simulink model "case33"  (R2014a)
settings: Solver=ode45  StartTime=0.0  StopTime=0.001  RelTol=1e-3
libraries: powerlib x143
(part 1 of 2)
settings Model: Creator=9502085  LastModifiedBy=9502085

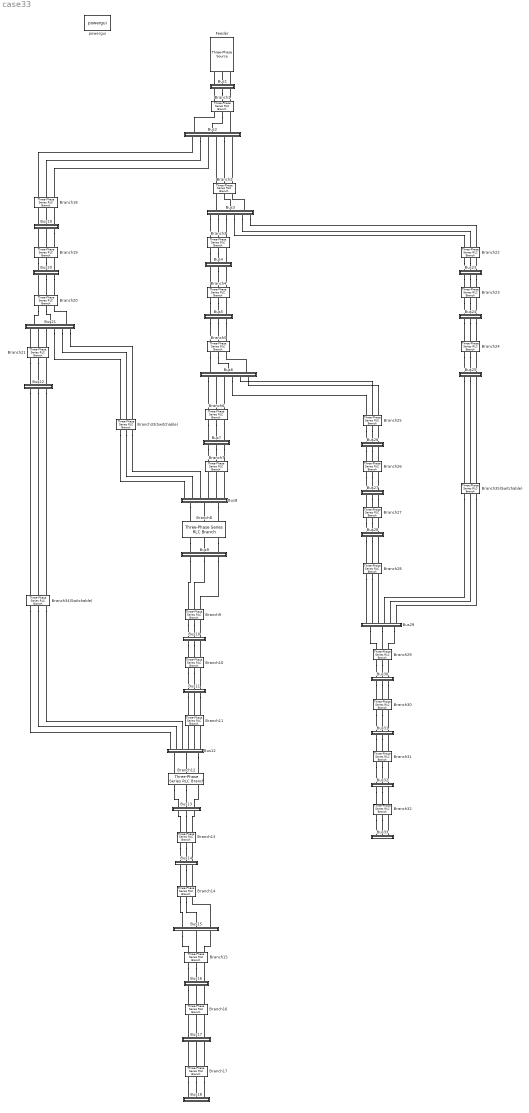
== system case33 ==
  " Branch26" : powerlib/Elements/Three-Phase Series RLC Branch  LConnTagsString=A|B|C  RConnTagsString=A|B|C  BranchType=RLC  Resistance=1  Inductance=1e-3  Capacitance=1e-6  Measurements=None
  Branch{1..25,27..32} (31 alike) : powerlib/Elements/Three-Phase Series RLC Branch  LConnTagsString=A|B|C  RConnTagsString=A|B|C  BranchType=RLC  Resistance=1  Inductance=1e-3  Capacitance=1e-6  Measurements=None
  Branch33(Switchable) : powerlib/Elements/Three-Phase Series RLC Branch  LConnTagsString=A|B|C  RConnTagsString=A|B|C  BranchType=RLC  Resistance=1  Inductance=1e-3  Capacitance=1e-6  Measurements=None
  Branch34(Switchable) : powerlib/Elements/Three-Phase Series RLC Branch  LConnTagsString=A|B|C  RConnTagsString=A|B|C  BranchType=RLC  Resistance=1  Inductance=1e-3  Capacitance=1e-6  Measurements=None
  Branch35(Switchable) : powerlib/Elements/Three-Phase Series RLC Branch  LConnTagsString=A|B|C  RConnTagsString=A|B|C  BranchType=RLC  Resistance=1  Inductance=1e-3  Capacitance=1e-6  Measurements=None
  Bus1 : Subsystem
  Bus10 : Subsystem
  Bus11 : Subsystem
  Bus12 : Subsystem
  Bus13 : Subsystem
  Bus14 : Subsystem
  Bus15 : Subsystem
  Bus16 : Subsystem
  Bus17 : Subsystem
  Bus18 : Subsystem
  Bus19 : Subsystem
  Bus2 : Subsystem
  Bus20 : Subsystem
  Bus21 : Subsystem
  Bus22 : Subsystem
  Bus23 : Subsystem
  Bus24 : Subsystem
  Bus25 : Subsystem
  Bus26 : Subsystem
  Bus27 : Subsystem
  Bus28 : Subsystem
  Bus29 : Subsystem
  Bus3 : Subsystem
  Bus30 : Subsystem
  Bus31 : Subsystem
  Bus32 : Subsystem
  Bus33 : Subsystem
  Bus4 : Subsystem
  Bus5 : Subsystem
  Bus6 : Subsystem
  Bus7 : Subsystem
  Bus8 : Subsystem
  Bus9 : Subsystem
  Feeder : powerlib/Electrical Sources/Three-Phase Source  Voltage=25e3  PhaseAngle=0  Frequency=60  InternalConnection=Yg  SpecifyImpedance=on  Resistance=0.8929  Inductance=16.58e-3  ShortCircuitLevel=100e6  BaseVoltage=25e3  XRratio=7  BusType=swing  Pref=0  Qref=0  Qmin=-inf  Qmax=inf
  powergui : powerlib/powergui  Priority=1  SimulationMode=Continuous  SolverType=Tustin  SampleTime=50e-6  frequency=60  SPID=off  DisableSnubberDevices=off  DisableRonSwitches=off  DisableVfSwitches=off  SwTol=0  Interpol=off  DisplayEquations=off  Ts=0  methode=off  frequencyindice=60  Pbase=100e6  ErrMax=1e-4  Iterations=50  UnitsV=kV  UnitsW=MW  FunctionMessages=off  echomessages=off  HookPort=off  EnableUseOfTLC=off  x0status=blocks  RestoreLinks=warning  ResistiveCurrentMeasurement=off  Frange=[0:2:500]  Ylog=off  Xlog=on  ShowGrid=off  save=off  variable=ZData  structure=0  ZoomFFT=off  StartTime=0.0  cycles=1  DisplayStyle=1  fundamental=60  FreqAxis=off  MaxFrequency=1000  frequencyindicesteady=1  RmsSteady=1  display=off
  connections:
  Bus1/RConn2 -- Branch1/LConn2
  Bus3/RConn2 -- Branch3/LConn2
  Bus3/RConn3 -- Branch3/LConn3
  Bus3/RConn1 -- Branch3/LConn1
  Bus4/RConn2 -- Branch4/LConn2
  Bus5/RConn2 -- Branch5/LConn2
  Bus5/RConn3 -- Branch5/LConn3
  Bus5/RConn1 -- Branch5/LConn1
  Branch6/LConn3 -- Bus6/RConn3
  Bus7/RConn3 -- Branch7/LConn3
  Bus9/RConn1 -- Branch9/LConn1
  Bus19/RConn3 -- Branch19/LConn3
  Bus20/RConn3 -- Branch20/LConn3
  Bus23/RConn3 -- Branch23/LConn3
  Bus27/RConn3 -- Branch27/LConn3
  Bus27/RConn2 -- Branch27/LConn2
  Branch33(Switchable)/RConn1 -- Bus8/LConn1
  Branch33(Switchable)/RConn2 -- Bus8/LConn2
  Branch33(Switchable)/RConn3 -- Bus8/LConn3
  Bus3/LConn1 -- Branch2/RConn1
  Bus3/LConn2 -- Branch2/RConn2
  Bus3/LConn3 -- Branch2/RConn3
  Bus19/LConn3 -- Branch18/RConn3
  Bus19/LConn2 -- Branch18/RConn2
  Bus19/LConn1 -- Branch18/RConn1
  Branch19/LConn1 -- Bus19/RConn1
  Branch19/LConn2 -- Bus19/RConn2
  Bus20/RConn2 -- Branch20/LConn2
  Bus20/LConn3 -- Branch19/RConn3
  Branch19/RConn2 -- Bus20/LConn2
  Branch19/RConn1 -- Bus20/LConn1
  Branch20/LConn1 -- Bus20/RConn1
  Branch20/RConn3 -- Bus21/LConn3
  Branch20/RConn2 -- Bus21/LConn2
  Branch20/RConn1 -- Bus21/LConn1
  Branch21/LConn1 -- Bus21/RConn1
  Branch21/LConn2 -- Bus21/RConn2
  Branch21/LConn3 -- Bus21/RConn3
  Bus22/LConn3 -- Branch21/RConn3
  Branch21/RConn1 -- Bus22/LConn1
  Bus22/RConn1 -- Branch34(Switchable)/LConn1
  Bus22/RConn2 -- Branch34(Switchable)/LConn2
  Bus22/RConn3 -- Branch34(Switchable)/LConn3
  Branch4/LConn3 -- Bus4/RConn3
  Bus4/LConn3 -- Branch3/RConn3
  Branch3/RConn2 -- Bus4/LConn2
  Branch3/RConn1 -- Bus4/LConn1
  Branch4/LConn1 -- Bus4/RConn1
  Bus2/LConn3 -- Branch1/RConn3
  Branch1/RConn2 -- Bus2/LConn2
  Bus2/LConn1 -- Branch1/RConn1
  Bus5/LConn3 -- Branch4/RConn3
  Branch4/RConn2 -- Bus5/LConn2
  Branch4/RConn1 -- Bus5/LConn1
  Bus6/LConn3 -- Branch5/RConn3
  Branch5/RConn2 -- Bus6/LConn2
  Branch5/RConn1 -- Bus6/LConn1
  Bus6/RConn1 -- Branch6/LConn1
  Branch6/LConn2 -- Bus6/RConn2
  Bus7/LConn3 -- Branch6/RConn3
  Branch6/RConn2 -- Bus7/LConn2
  Branch6/RConn1 -- Bus7/LConn1
  Bus7/RConn1 -- Branch7/LConn1
  Bus7/RConn2 -- Branch7/LConn2
  Branch8/RConn3 -- Bus9/LConn3
  Bus9/LConn2 -- Branch8/RConn2
  Branch8/RConn1 -- Bus9/LConn1
  Bus9/RConn2 -- Branch9/LConn2
  Bus9/RConn3 -- Branch9/LConn3
  Bus10/LConn3 -- Branch9/RConn3
  Branch9/RConn2 -- Bus10/LConn2
  Branch9/RConn1 -- Bus10/LConn1
  Bus10/RConn1 -- Branch10/LConn1
  Bus10/RConn2 -- Branch10/LConn2
  Branch10/LConn3 -- Bus10/RConn3
  Bus11/LConn3 -- Branch10/RConn3
  Bus11/RConn3 -- Branch11/LConn3
  Branch11/LConn2 -- Bus11/RConn2
  Bus11/RConn1 -- Branch11/LConn1
  Branch10/RConn1 -- Bus11/LConn1
  Branch10/RConn2 -- Bus11/LConn2
  Bus13/LConn3 -- Branch12/RConn3
  Bus13/RConn3 -- Branch13/LConn3
  Bus13/RConn2 -- Branch13/LConn2
  Branch12/RConn2 -- Bus13/LConn2
  Branch12/RConn1 -- Bus13/LConn1
  Bus13/RConn1 -- Branch13/LConn1
  Bus14/LConn3 -- Branch13/RConn3
  Branch14/LConn3 -- Bus14/RConn3
  Branch13/RConn2 -- Bus14/LConn2
  Branch13/RConn1 -- Bus14/LConn1
  Branch14/LConn1 -- Bus14/RConn1
  Bus14/RConn2 -- Branch14/LConn2
  Bus15/LConn3 -- Branch14/RConn3
  Branch14/RConn2 -- Bus15/LConn2
  Branch14/RConn1 -- Bus15/LConn1
  Bus16/LConn3 -- Branch15/RConn3
  Branch15/RConn2 -- Bus16/LConn2
  Branch15/RConn1 -- Bus16/LConn1
  Bus17/LConn3 -- Branch16/RConn3
  Bus17/LConn2 -- Branch16/RConn2
  Bus17/LConn1 -- Branch16/RConn1
  Branch17/RConn2 -- Bus18/LConn2
  Branch17/RConn1 -- Bus18/LConn1
  Bus23/LConn3 -- Branch22/RConn3
  Branch22/RConn2 -- Bus23/LConn2
  Branch22/RConn1 -- Bus23/LConn1
  Bus23/RConn1 -- Branch23/LConn1
  Bus23/RConn2 -- Branch23/LConn2
  Bus24/LConn3 -- Branch23/RConn3
  Bus24/RConn3 -- Branch24/LConn3
  Branch23/RConn2 -- Bus24/LConn2
  Branch23/RConn1 -- Bus24/LConn1
  Bus24/RConn1 -- Branch24/LConn1
  Bus24/RConn2 -- Branch24/LConn2
  Bus25/LConn3 -- Branch24/RConn3
  Branch35(Switchable)/LConn3 -- Bus25/RConn3
  Bus25/RConn2 -- Branch35(Switchable)/LConn2
  Bus25/RConn1 -- Branch35(Switchable)/LConn1
  Branch24/RConn1 -- Bus25/LConn1
  Branch24/RConn2 -- Bus25/LConn2
  Bus26/LConn3 -- Branch25/RConn3
  " Branch26"/LConn3 -- Bus26/RConn3
  Branch25/RConn2 -- Bus26/LConn2
  Branch25/RConn1 -- Bus26/LConn1
  Bus26/RConn1 -- " Branch26"/LConn1
  Bus26/RConn2 -- " Branch26"/LConn2
  Bus27/LConn3 -- " Branch26"/RConn3
  Branch27/LConn1 -- Bus27/RConn1
  " Branch26"/RConn1 -- Bus27/LConn1
  " Branch26"/RConn2 -- Bus27/LConn2
  Bus28/LConn3 -- Branch27/RConn3
  Branch27/RConn2 -- Bus28/LConn2
  Branch27/RConn1 -- Bus28/LConn1
  Branch28/LConn3 -- Bus28/RConn3
  Bus28/RConn2 -- Branch28/LConn2
  Bus28/RConn1 -- Branch28/LConn1
  Bus29/LConn3 -- Branch28/RConn3
  Branch28/RConn2 -- Bus29/LConn2
  Branch28/RConn1 -- Bus29/LConn1
  Bus29/RConn3 -- Branch29/LConn3
  Bus29/RConn2 -- Branch29/LConn2
  Bus29/RConn1 -- Branch29/LConn1
  Bus30/LConn3 -- Branch29/RConn3
  Branch29/RConn2 -- Bus30/LConn2
  Branch29/RConn1 -- Bus30/LConn1
  Bus30/RConn3 -- Branch30/LConn3
  Bus30/RConn2 -- Branch30/LConn2
  Bus30/RConn1 -- Branch30/LConn1
  Bus31/LConn3 -- Branch30/RConn3
  Branch31/LConn3 -- Bus31/RConn3
  Branch30/RConn2 -- Bus31/LConn2
  Branch30/RConn1 -- Bus31/LConn1
  Bus31/RConn2 -- Branch31/LConn2
  Bus31/RConn1 -- Branch31/LConn1
  Bus32/LConn3 -- Branch31/RConn3
  Branch31/RConn2 -- Bus32/LConn2
  Branch31/RConn1 -- Bus32/LConn1
  Branch32/LConn3 -- Bus32/RConn3
  Bus32/RConn2 -- Branch32/LConn2
  Bus32/RConn1 -- Branch32/LConn1
  Bus33/LConn3 -- Branch32/RConn3
  Branch32/RConn2 -- Bus33/LConn2
  Branch32/RConn1 -- Bus33/LConn1
  Branch17/RConn3 -- Bus18/LConn3
  Bus1/LConn2 -- Feeder/RConn2
  Bus1/LConn1 -- Feeder/RConn1
  Bus1/LConn3 -- Feeder/RConn3
  Branch1/LConn1 -- Bus1/RConn1
  Branch1/LConn3 -- Bus1/RConn3
  Bus6/RConn4 -- Branch25/LConn1
  Bus6/RConn5 -- Branch25/LConn2
  Bus6/RConn6 -- Branch25/LConn3
  Branch2/LConn3 -- Bus2/RConn6
  Bus2/RConn5 -- Branch2/LConn2
  Branch2/LConn1 -- Bus2/RConn4
  Branch18/LConn3 -- Bus2/RConn3
  Bus2/RConn2 -- Branch18/LConn2
  Branch18/LConn1 -- Bus2/RConn1
  Bus3/RConn4 -- Branch22/LConn1
  Bus3/RConn5 -- Branch22/LConn2
  Bus3/RConn6 -- Branch22/LConn3
  Bus8/LConn6 -- Branch7/RConn3
  Bus8/LConn4 -- Branch7/RConn1
  Bus8/LConn5 -- Branch7/RConn2
  Bus8/RConn1 -- Branch8/LConn1
  Branch8/LConn2 -- Bus8/RConn2
  Bus8/RConn3 -- Branch8/LConn3
  Bus21/RConn4 -- Branch33(Switchable)/LConn1
  Bus21/RConn5 -- Branch33(Switchable)/LConn2
  Bus21/RConn6 -- Branch33(Switchable)/LConn3
  Branch21/RConn2 -- Bus22/LConn2
  Bus12/LConn6 -- Branch11/RConn3
  Bus12/LConn5 -- Branch11/RConn2
  Bus12/LConn4 -- Branch11/RConn1
  Branch34(Switchable)/RConn3 -- Bus12/LConn3
  Branch34(Switchable)/RConn2 -- Bus12/LConn2
  Branch34(Switchable)/RConn1 -- Bus12/LConn1
  Branch12/LConn2 -- Bus12/RConn2
  Branch12/LConn1 -- Bus12/RConn1
  Bus12/RConn3 -- Branch12/LConn3
  Branch15/LConn2 -- Bus15/RConn2
  Bus15/RConn1 -- Branch15/LConn1
  Branch15/LConn3 -- Bus15/RConn3
  Branch16/LConn2 -- Bus16/RConn2
  Bus16/RConn1 -- Branch16/LConn1
  Branch16/LConn3 -- Bus16/RConn3
  Branch17/LConn3 -- Bus17/RConn3
  Branch17/LConn2 -- Bus17/RConn2
  Branch17/LConn1 -- Bus17/RConn1
  Branch35(Switchable)/RConn1 -- Bus29/LConn4
  Bus29/LConn5 -- Branch35(Switchable)/RConn2
  Branch35(Switchable)/RConn3 -- Bus29/LConn6

== system case33/Bus1 ==
  Bus1 : powerlib/Measurements/Three-Phase V-I Measurement  VoltageMeasurement=no  SetLabelV=off  LabelV=Vabc  Vpu=off  VpuLL=off  CurrentMeasurement=no  SetLabelI=off  LabelI=Iabc  Ipu=off  Pbase=100e6  Vbase=500e3  OutputType=Complex  PhasorSimulation=off  PSBequivalent=0
  CB1-2 : powerlib/Elements/Three-Phase Breaker  InitialState=open  SwitchA=on  SwitchB=on  SwitchC=on  SwitchTimes="[1/60  5/60]"  External=off  BreakerResistance=0.01  SnubberResistance=1e6  SnubberCapacitance=inf  Measurements=None
  InPhaseA : PMIOPort  Port=1  Side=Left
  InPhaseB : PMIOPort  Port=2  Side=Left
  InPhaseC : PMIOPort  Port=3  Side=Left
  OutPhaseA : PMIOPort  Port=4  Side=Right
  OutPhaseB : PMIOPort  Port=5  Side=Right
  OutPhaseC : PMIOPort  Port=6  Side=Right
  connections:
  CB1-2/LConn1 -- Bus1/RConn1
  CB1-2/RConn3 -- OutPhaseC/RConn1
  CB1-2/LConn2 -- Bus1/RConn2
  CB1-2/LConn3 -- Bus1/RConn3
  CB1-2/RConn1 -- OutPhaseA/RConn1
  CB1-2/RConn2 -- OutPhaseB/RConn1
  InPhaseA/RConn1 -- Bus1/LConn1
  InPhaseB/RConn1 -- Bus1/LConn2
  InPhaseC/RConn1 -- Bus1/LConn3

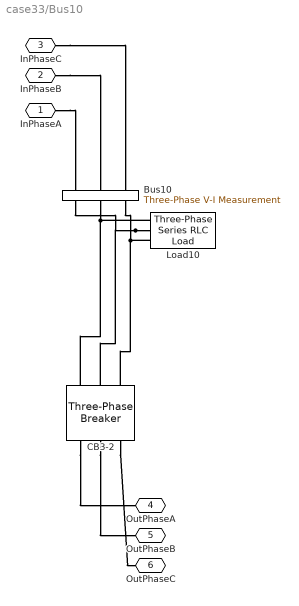
== system case33/Bus10 ==
  Bus10 : powerlib/Measurements/Three-Phase V-I Measurement  VoltageMeasurement=no  SetLabelV=off  LabelV=Vabc  Vpu=off  VpuLL=off  CurrentMeasurement=no  SetLabelI=off  LabelI=Iabc  Ipu=off  Pbase=100e6  Vbase=500e3  OutputType=Complex  PhasorSimulation=off  PSBequivalent=0
  CB3-2 : powerlib/Elements/Three-Phase Breaker  InitialState=open  SwitchA=on  SwitchB=on  SwitchC=on  SwitchTimes="[1/60  5/60]"  External=off  BreakerResistance=0.01  SnubberResistance=1e6  SnubberCapacitance=inf  Measurements=None
  Load10 : powerlib/Elements/Three-Phase Series RLC Load  LConnTagsString=A|B|C  Configuration=Y (grounded)  NominalVoltage=1000  NominalFrequency=60  ActivePower=10e3  InductivePower=100  CapacitivePower=100  Measurements=None  LoadType=constant Z
  InPhaseA : PMIOPort  Port=1  Side=Left
  InPhaseB : PMIOPort  Port=2  Side=Left
  InPhaseC : PMIOPort  Port=3  Side=Left
  OutPhaseA : PMIOPort  Port=4  Side=Right
  OutPhaseB : PMIOPort  Port=5  Side=Right
  OutPhaseC : PMIOPort  Port=6  Side=Right
  connections:
  Bus10/RConn1 -- CB3-2/LConn1 -- Load10/LConn1
  CB3-2/RConn3 -- OutPhaseC/RConn1
  Load10/LConn2 -- CB3-2/LConn2 -- Bus10/RConn2
  Load10/LConn3 -- CB3-2/LConn3 -- Bus10/RConn3
  CB3-2/RConn1 -- OutPhaseA/RConn1
  CB3-2/RConn2 -- OutPhaseB/RConn1
  InPhaseA/RConn1 -- Bus10/LConn1
  InPhaseB/RConn1 -- Bus10/LConn2
  InPhaseC/RConn1 -- Bus10/LConn3

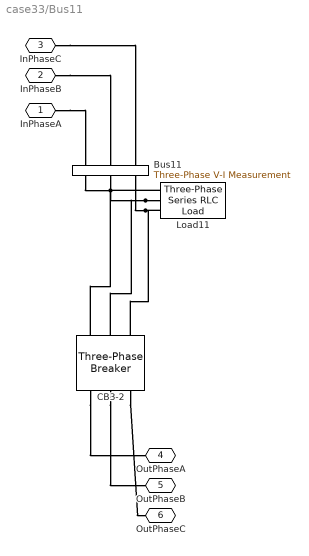
== system case33/Bus11 ==
  Bus11 : powerlib/Measurements/Three-Phase V-I Measurement  VoltageMeasurement=no  SetLabelV=off  LabelV=Vabc  Vpu=off  VpuLL=off  CurrentMeasurement=no  SetLabelI=off  LabelI=Iabc  Ipu=off  Pbase=100e6  Vbase=500e3  OutputType=Complex  PhasorSimulation=off  PSBequivalent=0
  CB3-2 : powerlib/Elements/Three-Phase Breaker  InitialState=open  SwitchA=on  SwitchB=on  SwitchC=on  SwitchTimes="[1/60  5/60]"  External=off  BreakerResistance=0.01  SnubberResistance=1e6  SnubberCapacitance=inf  Measurements=None
  Load11 : powerlib/Elements/Three-Phase Series RLC Load  LConnTagsString=A|B|C  Configuration=Y (grounded)  NominalVoltage=1000  NominalFrequency=60  ActivePower=10e3  InductivePower=100  CapacitivePower=100  Measurements=None  LoadType=constant Z
  InPhaseA : PMIOPort  Port=1  Side=Left
  InPhaseB : PMIOPort  Port=2  Side=Left
  InPhaseC : PMIOPort  Port=3  Side=Left
  OutPhaseA : PMIOPort  Port=4  Side=Right
  OutPhaseB : PMIOPort  Port=5  Side=Right
  OutPhaseC : PMIOPort  Port=6  Side=Right
  connections:
  Bus11/RConn1 -- CB3-2/LConn1 -- Load11/LConn1
  CB3-2/RConn3 -- OutPhaseC/RConn1
  Load11/LConn2 -- CB3-2/LConn2 -- Bus11/RConn2
  Bus11/RConn3 -- CB3-2/LConn3 -- Load11/LConn3
  CB3-2/RConn1 -- OutPhaseA/RConn1
  CB3-2/RConn2 -- OutPhaseB/RConn1
  InPhaseA/RConn1 -- Bus11/LConn1
  InPhaseB/RConn1 -- Bus11/LConn2
  InPhaseC/RConn1 -- Bus11/LConn3

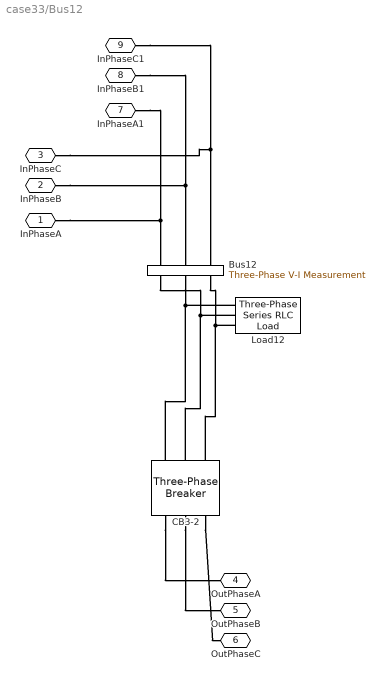
== system case33/Bus12 ==
  Bus12 : powerlib/Measurements/Three-Phase V-I Measurement  VoltageMeasurement=no  SetLabelV=off  LabelV=Vabc  Vpu=off  VpuLL=off  CurrentMeasurement=no  SetLabelI=off  LabelI=Iabc  Ipu=off  Pbase=100e6  Vbase=500e3  OutputType=Complex  PhasorSimulation=off  PSBequivalent=0
  CB3-2 : powerlib/Elements/Three-Phase Breaker  InitialState=open  SwitchA=on  SwitchB=on  SwitchC=on  SwitchTimes="[1/60  5/60]"  External=off  BreakerResistance=0.01  SnubberResistance=1e6  SnubberCapacitance=inf  Measurements=None
  Load12 : powerlib/Elements/Three-Phase Series RLC Load  LConnTagsString=A|B|C  Configuration=Y (grounded)  NominalVoltage=1000  NominalFrequency=60  ActivePower=10e3  InductivePower=100  CapacitivePower=100  Measurements=None  LoadType=constant Z
  InPhaseA : PMIOPort  Port=1  Side=Left
  InPhaseB : PMIOPort  Port=2  Side=Left
  InPhaseC : PMIOPort  Port=3  Side=Left
  OutPhaseA : PMIOPort  Port=4  Side=Right
  OutPhaseB : PMIOPort  Port=5  Side=Right
  OutPhaseC : PMIOPort  Port=6  Side=Right
  InPhaseA1 : PMIOPort  Port=7  Side=Left
  InPhaseB1 : PMIOPort  Port=8  Side=Left
  InPhaseC1 : PMIOPort  Port=9  Side=Left
  connections:
  Load12/LConn1 -- CB3-2/LConn1 -- Bus12/RConn1
  CB3-2/RConn3 -- OutPhaseC/RConn1
  Load12/LConn2 -- CB3-2/LConn2 -- Bus12/RConn2
  Load12/LConn3 -- CB3-2/LConn3 -- Bus12/RConn3
  CB3-2/RConn1 -- OutPhaseA/RConn1
  CB3-2/RConn2 -- OutPhaseB/RConn1
  InPhaseA1/RConn1 -- InPhaseA/RConn1 -- Bus12/LConn1
  InPhaseB1/RConn1 -- InPhaseB/RConn1 -- Bus12/LConn2
  InPhaseC1/RConn1 -- InPhaseC/RConn1 -- Bus12/LConn3

== system case33/Bus13 ==
  Bus13 : powerlib/Measurements/Three-Phase V-I Measurement  VoltageMeasurement=no  SetLabelV=off  LabelV=Vabc  Vpu=off  VpuLL=off  CurrentMeasurement=no  SetLabelI=off  LabelI=Iabc  Ipu=off  Pbase=100e6  Vbase=500e3  OutputType=Complex  PhasorSimulation=off  PSBequivalent=0
  CB3-2 : powerlib/Elements/Three-Phase Breaker  InitialState=open  SwitchA=on  SwitchB=on  SwitchC=on  SwitchTimes="[1/60  5/60]"  External=off  BreakerResistance=0.01  SnubberResistance=1e6  SnubberCapacitance=inf  Measurements=None
  Load13 : powerlib/Elements/Three-Phase Series RLC Load  LConnTagsString=A|B|C  Configuration=Y (grounded)  NominalVoltage=1000  NominalFrequency=60  ActivePower=10e3  InductivePower=100  CapacitivePower=100  Measurements=None  LoadType=constant Z
  InPhaseA : PMIOPort  Port=1  Side=Left
  InPhaseB : PMIOPort  Port=2  Side=Left
  InPhaseC : PMIOPort  Port=3  Side=Left
  OutPhaseA : PMIOPort  Port=4  Side=Right
  OutPhaseB : PMIOPort  Port=5  Side=Right
  OutPhaseC : PMIOPort  Port=6  Side=Right
  connections:
  Load13/LConn1 -- CB3-2/LConn1 -- Bus13/RConn1
  CB3-2/RConn3 -- OutPhaseC/RConn1
  Load13/LConn2 -- CB3-2/LConn2 -- Bus13/RConn2
  Bus13/RConn3 -- CB3-2/LConn3 -- Load13/LConn3
  CB3-2/RConn1 -- OutPhaseA/RConn1
  CB3-2/RConn2 -- OutPhaseB/RConn1
  InPhaseB/RConn1 -- Bus13/LConn2
  Bus13/LConn1 -- InPhaseA/RConn1
  InPhaseC/RConn1 -- Bus13/LConn3

== system case33/Bus14 ==
  Bus14 : powerlib/Measurements/Three-Phase V-I Measurement  VoltageMeasurement=no  SetLabelV=off  LabelV=Vabc  Vpu=off  VpuLL=off  CurrentMeasurement=no  SetLabelI=off  LabelI=Iabc  Ipu=off  Pbase=100e6  Vbase=500e3  OutputType=Complex  PhasorSimulation=off  PSBequivalent=0
  CB3-2 : powerlib/Elements/Three-Phase Breaker  InitialState=open  SwitchA=on  SwitchB=on  SwitchC=on  SwitchTimes="[1/60  5/60]"  External=off  BreakerResistance=0.01  SnubberResistance=1e6  SnubberCapacitance=inf  Measurements=None
  Load14 : powerlib/Elements/Three-Phase Series RLC Load  LConnTagsString=A|B|C  Configuration=Y (grounded)  NominalVoltage=1000  NominalFrequency=60  ActivePower=10e3  InductivePower=100  CapacitivePower=100  Measurements=None  LoadType=constant Z
  InPhaseA : PMIOPort  Port=1  Side=Left
  InPhaseB : PMIOPort  Port=2  Side=Left
  InPhaseC : PMIOPort  Port=3  Side=Left
  OutPhaseA : PMIOPort  Port=4  Side=Right
  OutPhaseB : PMIOPort  Port=5  Side=Right
  OutPhaseC : PMIOPort  Port=6  Side=Right
  connections:
  Bus14/RConn1 -- CB3-2/LConn1 -- Load14/LConn1
  CB3-2/RConn3 -- OutPhaseC/RConn1
  Load14/LConn2 -- CB3-2/LConn2 -- Bus14/RConn2
  Bus14/RConn3 -- CB3-2/LConn3 -- Load14/LConn3
  CB3-2/RConn1 -- OutPhaseA/RConn1
  CB3-2/RConn2 -- OutPhaseB/RConn1
  InPhaseB/RConn1 -- Bus14/LConn2
  InPhaseA/RConn1 -- Bus14/LConn1
  InPhaseC/RConn1 -- Bus14/LConn3

== system case33/Bus15 ==
  Bus15 : powerlib/Measurements/Three-Phase V-I Measurement  VoltageMeasurement=no  SetLabelV=off  LabelV=Vabc  Vpu=off  VpuLL=off  CurrentMeasurement=no  SetLabelI=off  LabelI=Iabc  Ipu=off  Pbase=100e6  Vbase=500e3  OutputType=Complex  PhasorSimulation=off  PSBequivalent=0
  CB3-2 : powerlib/Elements/Three-Phase Breaker  InitialState=open  SwitchA=on  SwitchB=on  SwitchC=on  SwitchTimes="[1/60  5/60]"  External=off  BreakerResistance=0.01  SnubberResistance=1e6  SnubberCapacitance=inf  Measurements=None
  Load15 : powerlib/Elements/Three-Phase Series RLC Load  LConnTagsString=A|B|C  Configuration=Y (grounded)  NominalVoltage=1000  NominalFrequency=60  ActivePower=10e3  InductivePower=100  CapacitivePower=100  Measurements=None  LoadType=constant Z
  InPhaseA : PMIOPort  Port=1  Side=Left
  InPhaseB : PMIOPort  Port=2  Side=Left
  InPhaseC : PMIOPort  Port=3  Side=Left
  OutPhaseA : PMIOPort  Port=4  Side=Right
  OutPhaseB : PMIOPort  Port=5  Side=Right
  OutPhaseC : PMIOPort  Port=6  Side=Right
  connections:
  Load15/LConn1 -- CB3-2/LConn1 -- Bus15/RConn1
  CB3-2/RConn3 -- OutPhaseC/RConn1
  Load15/LConn2 -- CB3-2/LConn2 -- Bus15/RConn2
  Load15/LConn3 -- CB3-2/LConn3 -- Bus15/RConn3
  CB3-2/RConn1 -- OutPhaseA/RConn1
  CB3-2/RConn2 -- OutPhaseB/RConn1
  InPhaseA/RConn1 -- Bus15/LConn1
  InPhaseB/RConn1 -- Bus15/LConn2
  InPhaseC/RConn1 -- Bus15/LConn3

== system case33/Bus16 ==
  Bus16 : powerlib/Measurements/Three-Phase V-I Measurement  VoltageMeasurement=no  SetLabelV=off  LabelV=Vabc  Vpu=off  VpuLL=off  CurrentMeasurement=no  SetLabelI=off  LabelI=Iabc  Ipu=off  Pbase=100e6  Vbase=500e3  OutputType=Complex  PhasorSimulation=off  PSBequivalent=0
  CB3-2 : powerlib/Elements/Three-Phase Breaker  InitialState=open  SwitchA=on  SwitchB=on  SwitchC=on  SwitchTimes="[1/60  5/60]"  External=off  BreakerResistance=0.01  SnubberResistance=1e6  SnubberCapacitance=inf  Measurements=None
  Load16 : powerlib/Elements/Three-Phase Series RLC Load  LConnTagsString=A|B|C  Configuration=Y (grounded)  NominalVoltage=1000  NominalFrequency=60  ActivePower=10e3  InductivePower=100  CapacitivePower=100  Measurements=None  LoadType=constant Z
  InPhaseA : PMIOPort  Port=1  Side=Left
  InPhaseB : PMIOPort  Port=2  Side=Left
  InPhaseC : PMIOPort  Port=3  Side=Left
  OutPhaseA : PMIOPort  Port=4  Side=Right
  OutPhaseB : PMIOPort  Port=5  Side=Right
  OutPhaseC : PMIOPort  Port=6  Side=Right
  connections:
  Bus16/RConn1 -- CB3-2/LConn1 -- Load16/LConn1
  CB3-2/RConn3 -- OutPhaseC/RConn1
  Load16/LConn2 -- CB3-2/LConn2 -- Bus16/RConn2
  Load16/LConn3 -- CB3-2/LConn3 -- Bus16/RConn3
  CB3-2/RConn1 -- OutPhaseA/RConn1
  CB3-2/RConn2 -- OutPhaseB/RConn1
  InPhaseC/RConn1 -- Bus16/LConn3
  InPhaseB/RConn1 -- Bus16/LConn2
  InPhaseA/RConn1 -- Bus16/LConn1

== system case33/Bus17 ==
  Bus17 : powerlib/Measurements/Three-Phase V-I Measurement  VoltageMeasurement=no  SetLabelV=off  LabelV=Vabc  Vpu=off  VpuLL=off  CurrentMeasurement=no  SetLabelI=off  LabelI=Iabc  Ipu=off  Pbase=100e6  Vbase=500e3  OutputType=Complex  PhasorSimulation=off  PSBequivalent=0
  CB3-2 : powerlib/Elements/Three-Phase Breaker  InitialState=open  SwitchA=on  SwitchB=on  SwitchC=on  SwitchTimes="[1/60  5/60]"  External=off  BreakerResistance=0.01  SnubberResistance=1e6  SnubberCapacitance=inf  Measurements=None
  Load17 : powerlib/Elements/Three-Phase Series RLC Load  LConnTagsString=A|B|C  Configuration=Y (grounded)  NominalVoltage=1000  NominalFrequency=60  ActivePower=10e3  InductivePower=100  CapacitivePower=100  Measurements=None  LoadType=constant Z
  InPhaseA : PMIOPort  Port=1  Side=Left
  InPhaseB : PMIOPort  Port=2  Side=Left
  InPhaseC : PMIOPort  Port=3  Side=Left
  OutPhaseA : PMIOPort  Port=4  Side=Right
  OutPhaseB : PMIOPort  Port=5  Side=Right
  OutPhaseC : PMIOPort  Port=6  Side=Right
  connections:
  Bus17/RConn1 -- CB3-2/LConn1 -- Load17/LConn1
  CB3-2/RConn3 -- OutPhaseC/RConn1
  Load17/LConn2 -- CB3-2/LConn2 -- Bus17/RConn2
  Bus17/RConn3 -- CB3-2/LConn3 -- Load17/LConn3
  CB3-2/RConn1 -- OutPhaseA/RConn1
  CB3-2/RConn2 -- OutPhaseB/RConn1
  InPhaseA/RConn1 -- Bus17/LConn1
  InPhaseB/RConn1 -- Bus17/LConn2
  InPhaseC/RConn1 -- Bus17/LConn3

== system case33/Bus18 ==
  Bus18 : powerlib/Measurements/Three-Phase V-I Measurement  VoltageMeasurement=no  SetLabelV=off  LabelV=Vabc  Vpu=off  VpuLL=off  CurrentMeasurement=no  SetLabelI=off  LabelI=Iabc  Ipu=off  Pbase=100e6  Vbase=500e3  OutputType=Complex  PhasorSimulation=off  PSBequivalent=0
  Capacitor18 : powerlib/Elements/Three-Phase Series RLC Load  LConnTagsString=A|B|C  Configuration=Y (grounded)  NominalVoltage=1000  NominalFrequency=60  ActivePower=0  InductivePower=0  CapacitivePower=400000  Measurements=None  LoadType=constant Z
  DG18 : powerlib/Electrical Sources/Three-Phase Source  Voltage=25e3  PhaseAngle=0  Frequency=60  InternalConnection=Yg  SpecifyImpedance=on  Resistance=0.8929  Inductance=16.58e-3  ShortCircuitLevel=100e6  BaseVoltage=25e3  XRratio=7  BusType=PV  Pref=200000  Qref=0  Qmin=-inf  Qmax=inf
  Load18 : powerlib/Elements/Three-Phase Series RLC Load  LConnTagsString=A|B|C  Configuration=Y (grounded)  NominalVoltage=1000  NominalFrequency=60  ActivePower=10e3  InductivePower=100  CapacitivePower=100  Measurements=None  LoadType=constant Z
  InPhaseA : PMIOPort  Port=1  Side=Left
  InPhaseB : PMIOPort  Port=2  Side=Left
  InPhaseC : PMIOPort  Port=3  Side=Left
  connections:
  Load18/LConn1 -- DG18/RConn1 -- Bus18/RConn1 -- Capacitor18/LConn1
  Bus18/RConn2 -- Capacitor18/LConn2 -- DG18/RConn2 -- Load18/LConn2
  Bus18/RConn3 -- Capacitor18/LConn3 -- DG18/RConn3 -- Load18/LConn3
  InPhaseA/RConn1 -- Bus18/LConn1
  InPhaseB/RConn1 -- Bus18/LConn2
  InPhaseC/RConn1 -- Bus18/LConn3

== system case33/Bus19 ==
  Bus19 : powerlib/Measurements/Three-Phase V-I Measurement  VoltageMeasurement=no  SetLabelV=off  LabelV=Vabc  Vpu=off  VpuLL=off  CurrentMeasurement=no  SetLabelI=off  LabelI=Iabc  Ipu=off  Pbase=100e6  Vbase=500e3  OutputType=Complex  PhasorSimulation=off  PSBequivalent=0
  CB3-2 : powerlib/Elements/Three-Phase Breaker  InitialState=open  SwitchA=on  SwitchB=on  SwitchC=on  SwitchTimes="[1/60  5/60]"  External=off  BreakerResistance=0.01  SnubberResistance=1e6  SnubberCapacitance=inf  Measurements=None
  Load19 : powerlib/Elements/Three-Phase Series RLC Load  LConnTagsString=A|B|C  Configuration=Y (grounded)  NominalVoltage=1000  NominalFrequency=60  ActivePower=10e3  InductivePower=100  CapacitivePower=100  Measurements=None  LoadType=constant Z
  InPhaseA : PMIOPort  Port=1  Side=Left
  InPhaseB : PMIOPort  Port=2  Side=Left
  InPhaseC : PMIOPort  Port=3  Side=Left
  OutPhaseA : PMIOPort  Port=4  Side=Right
  OutPhaseB : PMIOPort  Port=5  Side=Right
  OutPhaseC : PMIOPort  Port=6  Side=Right
  connections:
  Bus19/RConn1 -- CB3-2/LConn1 -- Load19/LConn1
  CB3-2/RConn3 -- OutPhaseC/RConn1
  Load19/LConn2 -- CB3-2/LConn2 -- Bus19/RConn2
  Bus19/RConn3 -- CB3-2/LConn3 -- Load19/LConn3
  CB3-2/RConn1 -- OutPhaseA/RConn1
  CB3-2/RConn2 -- OutPhaseB/RConn1
  Bus19/LConn1 -- InPhaseA/RConn1
  InPhaseB/RConn1 -- Bus19/LConn2
  InPhaseC/RConn1 -- Bus19/LConn3

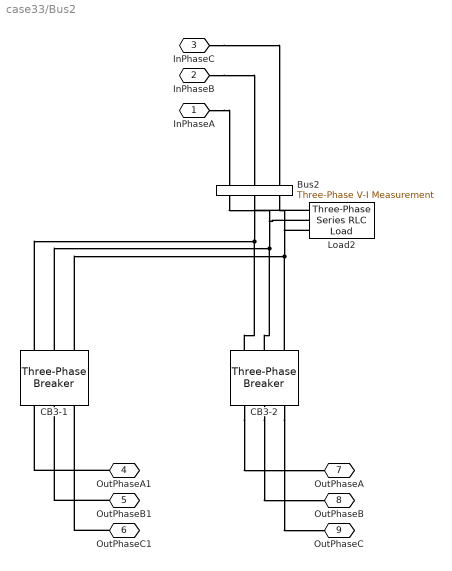
== system case33/Bus2 ==
  Bus2 : powerlib/Measurements/Three-Phase V-I Measurement  VoltageMeasurement=no  SetLabelV=off  LabelV=Vabc  Vpu=off  VpuLL=off  CurrentMeasurement=no  SetLabelI=off  LabelI=Iabc  Ipu=off  Pbase=100e6  Vbase=500e3  OutputType=Complex  PhasorSimulation=off  PSBequivalent=0
  CB3-1 : powerlib/Elements/Three-Phase Breaker  InitialState=open  SwitchA=on  SwitchB=on  SwitchC=on  SwitchTimes="[1/60  5/60]"  External=off  BreakerResistance=0.01  SnubberResistance=1e6  SnubberCapacitance=inf  Measurements=None
  CB3-2 : powerlib/Elements/Three-Phase Breaker  InitialState=open  SwitchA=on  SwitchB=on  SwitchC=on  SwitchTimes="[1/60  5/60]"  External=off  BreakerResistance=0.01  SnubberResistance=1e6  SnubberCapacitance=inf  Measurements=None
  Load2 : powerlib/Elements/Three-Phase Series RLC Load  LConnTagsString=A|B|C  Configuration=Y (grounded)  NominalVoltage=1000  NominalFrequency=60  ActivePower=10e3  InductivePower=100  CapacitivePower=100  Measurements=None  LoadType=constant Z
  InPhaseA : PMIOPort  Port=1  Side=Left
  InPhaseB : PMIOPort  Port=2  Side=Left
  InPhaseC : PMIOPort  Port=3  Side=Left
  OutPhaseA1 : PMIOPort  Port=4  Side=Right
  OutPhaseB1 : PMIOPort  Port=5  Side=Right
  OutPhaseC1 : PMIOPort  Port=6  Side=Right
  OutPhaseA : PMIOPort  Port=7  Side=Right
  OutPhaseB : PMIOPort  Port=8  Side=Right
  OutPhaseC : PMIOPort  Port=9  Side=Right
  connections:
  CB3-1/LConn1 -- CB3-2/LConn1 -- Load2/LConn1 -- Bus2/RConn1
  CB3-1/LConn2 -- Load2/LConn2 -- Bus2/RConn2 -- CB3-2/LConn2
  CB3-1/LConn3 -- Load2/LConn3 -- Bus2/RConn3 -- CB3-2/LConn3
  InPhaseC/RConn1 -- Bus2/LConn3
  InPhaseB/RConn1 -- Bus2/LConn2
  InPhaseA/RConn1 -- Bus2/LConn1
  OutPhaseA1/RConn1 -- CB3-1/RConn1
  OutPhaseC1/RConn1 -- CB3-1/RConn3
  OutPhaseB1/RConn1 -- CB3-1/RConn2
  CB3-2/RConn1 -- OutPhaseA/RConn1
  CB3-2/RConn2 -- OutPhaseB/RConn1
  CB3-2/RConn3 -- OutPhaseC/RConn1

== system case33/Bus20 ==
  Bus20 : powerlib/Measurements/Three-Phase V-I Measurement  VoltageMeasurement=no  SetLabelV=off  LabelV=Vabc  Vpu=off  VpuLL=off  CurrentMeasurement=no  SetLabelI=off  LabelI=Iabc  Ipu=off  Pbase=100e6  Vbase=500e3  OutputType=Complex  PhasorSimulation=off  PSBequivalent=0
  CB3-2 : powerlib/Elements/Three-Phase Breaker  InitialState=open  SwitchA=on  SwitchB=on  SwitchC=on  SwitchTimes="[1/60  5/60]"  External=off  BreakerResistance=0.01  SnubberResistance=1e6  SnubberCapacitance=inf  Measurements=None
  Load20 : powerlib/Elements/Three-Phase Series RLC Load  LConnTagsString=A|B|C  Configuration=Y (grounded)  NominalVoltage=1000  NominalFrequency=60  ActivePower=10e3  InductivePower=100  CapacitivePower=100  Measurements=None  LoadType=constant Z
  InPhaseA : PMIOPort  Port=1  Side=Left
  InPhaseB : PMIOPort  Port=2  Side=Left
  InPhaseC : PMIOPort  Port=3  Side=Left
  OutPhaseA : PMIOPort  Port=4  Side=Right
  OutPhaseB : PMIOPort  Port=5  Side=Right
  OutPhaseC : PMIOPort  Port=6  Side=Right
  connections:
  Bus20/RConn1 -- CB3-2/LConn1 -- Load20/LConn1
  CB3-2/RConn3 -- OutPhaseC/RConn1
  Load20/LConn2 -- CB3-2/LConn2 -- Bus20/RConn2
  Bus20/RConn3 -- CB3-2/LConn3 -- Load20/LConn3
  CB3-2/RConn1 -- OutPhaseA/RConn1
  CB3-2/RConn2 -- OutPhaseB/RConn1
  InPhaseA/RConn1 -- Bus20/LConn1
  InPhaseB/RConn1 -- Bus20/LConn2
  InPhaseC/RConn1 -- Bus20/LConn3

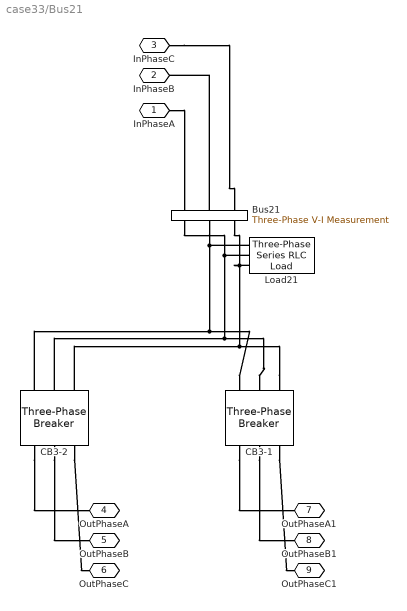
== system case33/Bus21 ==
  Bus21 : powerlib/Measurements/Three-Phase V-I Measurement  VoltageMeasurement=no  SetLabelV=off  LabelV=Vabc  Vpu=off  VpuLL=off  CurrentMeasurement=no  SetLabelI=off  LabelI=Iabc  Ipu=off  Pbase=100e6  Vbase=500e3  OutputType=Complex  PhasorSimulation=off  PSBequivalent=0
  CB3-1 : powerlib/Elements/Three-Phase Breaker  InitialState=open  SwitchA=on  SwitchB=on  SwitchC=on  SwitchTimes="[1/60  5/60]"  External=off  BreakerResistance=0.01  SnubberResistance=1e6  SnubberCapacitance=inf  Measurements=None
  CB3-2 : powerlib/Elements/Three-Phase Breaker  InitialState=open  SwitchA=on  SwitchB=on  SwitchC=on  SwitchTimes="[1/60  5/60]"  External=off  BreakerResistance=0.01  SnubberResistance=1e6  SnubberCapacitance=inf  Measurements=None
  Load21 : powerlib/Elements/Three-Phase Series RLC Load  LConnTagsString=A|B|C  Configuration=Y (grounded)  NominalVoltage=1000  NominalFrequency=60  ActivePower=10e3  InductivePower=100  CapacitivePower=100  Measurements=None  LoadType=constant Z
  InPhaseA : PMIOPort  Port=1  Side=Left
  InPhaseB : PMIOPort  Port=2  Side=Left
  InPhaseC : PMIOPort  Port=3  Side=Left
  OutPhaseA : PMIOPort  Port=4  Side=Right
  OutPhaseB : PMIOPort  Port=5  Side=Right
  OutPhaseC : PMIOPort  Port=6  Side=Right
  OutPhaseA1 : PMIOPort  Port=7  Side=Right
  OutPhaseB1 : PMIOPort  Port=8  Side=Right
  OutPhaseC1 : PMIOPort  Port=9  Side=Right
  connections:
  CB3-1/LConn1 -- Load21/LConn1 -- Bus21/RConn1 -- CB3-2/LConn1
  CB3-2/RConn3 -- OutPhaseC/RConn1
  CB3-1/LConn2 -- Load21/LConn2 -- Bus21/RConn2 -- CB3-2/LConn2
  CB3-1/LConn3 -- Bus21/RConn3 -- Load21/LConn3 -- CB3-2/LConn3
  CB3-2/RConn1 -- OutPhaseA/RConn1
  CB3-2/RConn2 -- OutPhaseB/RConn1
  InPhaseA/RConn1 -- Bus21/LConn1
  Bus21/LConn2 -- InPhaseB/RConn1
  InPhaseC/RConn1 -- Bus21/LConn3
  CB3-1/RConn3 -- OutPhaseC1/RConn1
  CB3-1/RConn1 -- OutPhaseA1/RConn1
  CB3-1/RConn2 -- OutPhaseB1/RConn1

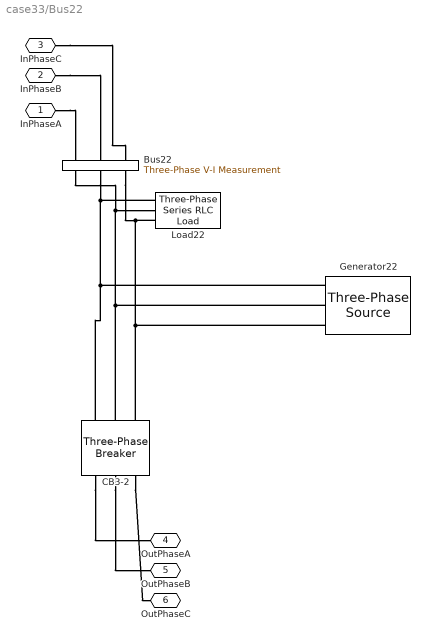
== system case33/Bus22 ==
  Bus22 : powerlib/Measurements/Three-Phase V-I Measurement  VoltageMeasurement=no  SetLabelV=off  LabelV=Vabc  Vpu=off  VpuLL=off  CurrentMeasurement=no  SetLabelI=off  LabelI=Iabc  Ipu=off  Pbase=100e6  Vbase=500e3  OutputType=Complex  PhasorSimulation=off  PSBequivalent=0
  CB3-2 : powerlib/Elements/Three-Phase Breaker  InitialState=open  SwitchA=on  SwitchB=on  SwitchC=on  SwitchTimes="[1/60  5/60]"  External=off  BreakerResistance=0.01  SnubberResistance=1e6  SnubberCapacitance=inf  Measurements=None
  Generator22 : powerlib/Electrical Sources/Three-Phase Source  Voltage=25e3  PhaseAngle=0  Frequency=60  InternalConnection=Yg  SpecifyImpedance=on  Resistance=0.8929  Inductance=16.58e-3  ShortCircuitLevel=100e6  BaseVoltage=25e3  XRratio=7  BusType=PV  Pref=200000  Qref=0  Qmin=-inf  Qmax=inf
  Load22 : powerlib/Elements/Three-Phase Series RLC Load  LConnTagsString=A|B|C  Configuration=Y (grounded)  NominalVoltage=1000  NominalFrequency=60  ActivePower=10e3  InductivePower=100  CapacitivePower=100  Measurements=None  LoadType=constant Z
  InPhaseA : PMIOPort  Port=1  Side=Left
  InPhaseB : PMIOPort  Port=2  Side=Left
  InPhaseC : PMIOPort  Port=3  Side=Left
  OutPhaseA : PMIOPort  Port=4  Side=Right
  OutPhaseB : PMIOPort  Port=5  Side=Right
  OutPhaseC : PMIOPort  Port=6  Side=Right
  connections:
  CB3-2/RConn3 -- OutPhaseC/RConn1
  Bus22/RConn2 -- Generator22/RConn2 -- CB3-2/LConn2 -- Load22/LConn2
  Bus22/RConn3 -- Generator22/RConn3 -- CB3-2/LConn3 -- Load22/LConn3
  CB3-2/RConn1 -- OutPhaseA/RConn1
  CB3-2/RConn2 -- OutPhaseB/RConn1
  Load22/LConn1 -- Generator22/RConn1 -- CB3-2/LConn1 -- Bus22/RConn1
  InPhaseA/RConn1 -- Bus22/LConn1
  InPhaseB/RConn1 -- Bus22/LConn2
  InPhaseC/RConn1 -- Bus22/LConn3

== system case33/Bus23 ==
  Bus23 : powerlib/Measurements/Three-Phase V-I Measurement  VoltageMeasurement=no  SetLabelV=off  LabelV=Vabc  Vpu=off  VpuLL=off  CurrentMeasurement=no  SetLabelI=off  LabelI=Iabc  Ipu=off  Pbase=100e6  Vbase=500e3  OutputType=Complex  PhasorSimulation=off  PSBequivalent=0
  CB3-2 : powerlib/Elements/Three-Phase Breaker  InitialState=open  SwitchA=on  SwitchB=on  SwitchC=on  SwitchTimes="[1/60  5/60]"  External=off  BreakerResistance=0.01  SnubberResistance=1e6  SnubberCapacitance=inf  Measurements=None
  Load23 : powerlib/Elements/Three-Phase Series RLC Load  LConnTagsString=A|B|C  Configuration=Y (grounded)  NominalVoltage=1000  NominalFrequency=60  ActivePower=10e3  InductivePower=100  CapacitivePower=100  Measurements=None  LoadType=constant Z
  InPhaseA : PMIOPort  Port=1  Side=Left
  InPhaseB : PMIOPort  Port=2  Side=Left
  InPhaseC : PMIOPort  Port=3  Side=Left
  OutPhaseA : PMIOPort  Port=4  Side=Right
  OutPhaseB : PMIOPort  Port=5  Side=Right
  OutPhaseC : PMIOPort  Port=6  Side=Right
  connections:
  Bus23/RConn1 -- CB3-2/LConn1 -- Load23/LConn1
  CB3-2/RConn3 -- OutPhaseC/RConn1
  Load23/LConn2 -- CB3-2/LConn2 -- Bus23/RConn2
  Load23/LConn3 -- CB3-2/LConn3 -- Bus23/RConn3
  CB3-2/RConn1 -- OutPhaseA/RConn1
  CB3-2/RConn2 -- OutPhaseB/RConn1
  InPhaseA/RConn1 -- Bus23/LConn1
  InPhaseB/RConn1 -- Bus23/LConn2
  InPhaseC/RConn1 -- Bus23/LConn3

== system case33/Bus24 ==
  Bus24 : powerlib/Measurements/Three-Phase V-I Measurement  VoltageMeasurement=no  SetLabelV=off  LabelV=Vabc  Vpu=off  VpuLL=off  CurrentMeasurement=no  SetLabelI=off  LabelI=Iabc  Ipu=off  Pbase=100e6  Vbase=500e3  OutputType=Complex  PhasorSimulation=off  PSBequivalent=0
  CB3-2 : powerlib/Elements/Three-Phase Breaker  InitialState=open  SwitchA=on  SwitchB=on  SwitchC=on  SwitchTimes="[1/60  5/60]"  External=off  BreakerResistance=0.01  SnubberResistance=1e6  SnubberCapacitance=inf  Measurements=None
  Load24 : powerlib/Elements/Three-Phase Series RLC Load  LConnTagsString=A|B|C  Configuration=Y (grounded)  NominalVoltage=1000  NominalFrequency=60  ActivePower=10e3  InductivePower=100  CapacitivePower=100  Measurements=None  LoadType=constant Z
  InPhaseA : PMIOPort  Port=1  Side=Left
  InPhaseB : PMIOPort  Port=2  Side=Left
  InPhaseC : PMIOPort  Port=3  Side=Left
  OutPhaseA : PMIOPort  Port=4  Side=Right
  OutPhaseB : PMIOPort  Port=5  Side=Right
  OutPhaseC : PMIOPort  Port=6  Side=Right
  connections:
  Bus24/RConn1 -- CB3-2/LConn1 -- Load24/LConn1
  CB3-2/RConn3 -- OutPhaseC/RConn1
  Load24/LConn2 -- CB3-2/LConn2 -- Bus24/RConn2
  Load24/LConn3 -- CB3-2/LConn3 -- Bus24/RConn3
  CB3-2/RConn1 -- OutPhaseA/RConn1
  CB3-2/RConn2 -- OutPhaseB/RConn1
  InPhaseA/RConn1 -- Bus24/LConn1
  InPhaseB/RConn1 -- Bus24/LConn2
  InPhaseC/RConn1 -- Bus24/LConn3

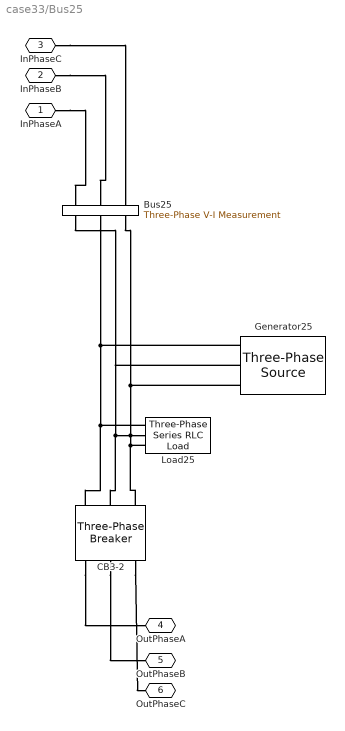
== system case33/Bus25 ==
  Bus25 : powerlib/Measurements/Three-Phase V-I Measurement  VoltageMeasurement=no  SetLabelV=off  LabelV=Vabc  Vpu=off  VpuLL=off  CurrentMeasurement=no  SetLabelI=off  LabelI=Iabc  Ipu=off  Pbase=100e6  Vbase=500e3  OutputType=Complex  PhasorSimulation=off  PSBequivalent=0
  CB3-2 : powerlib/Elements/Three-Phase Breaker  InitialState=open  SwitchA=on  SwitchB=on  SwitchC=on  SwitchTimes="[1/60  5/60]"  External=off  BreakerResistance=0.01  SnubberResistance=1e6  SnubberCapacitance=inf  Measurements=None
  Generator25 : powerlib/Electrical Sources/Three-Phase Source  Voltage=25e3  PhaseAngle=0  Frequency=60  InternalConnection=Yg  SpecifyImpedance=on  Resistance=0.8929  Inductance=16.58e-3  ShortCircuitLevel=100e6  BaseVoltage=25e3  XRratio=7  BusType=PV  Pref=200000  Qref=0  Qmin=-inf  Qmax=inf
  Load25 : powerlib/Elements/Three-Phase Series RLC Load  LConnTagsString=A|B|C  Configuration=Y (grounded)  NominalVoltage=1000  NominalFrequency=60  ActivePower=10e3  InductivePower=100  CapacitivePower=100  Measurements=None  LoadType=constant Z
  InPhaseA : PMIOPort  Port=1  Side=Left
  InPhaseB : PMIOPort  Port=2  Side=Left
  InPhaseC : PMIOPort  Port=3  Side=Left
  OutPhaseA : PMIOPort  Port=4  Side=Right
  OutPhaseB : PMIOPort  Port=5  Side=Right
  OutPhaseC : PMIOPort  Port=6  Side=Right
  connections:
  Bus25/RConn1 -- Generator25/RConn1 -- CB3-2/LConn1 -- Load25/LConn1
  CB3-2/RConn3 -- OutPhaseC/RConn1
  Load25/LConn2 -- CB3-2/LConn2 -- Bus25/RConn2 -- Generator25/RConn2
  Bus25/RConn3 -- Generator25/RConn3 -- CB3-2/LConn3 -- Load25/LConn3
  CB3-2/RConn1 -- OutPhaseA/RConn1
  CB3-2/RConn2 -- OutPhaseB/RConn1
  InPhaseB/RConn1 -- Bus25/LConn2
  InPhaseA/RConn1 -- Bus25/LConn1
  InPhaseC/RConn1 -- Bus25/LConn3

== system case33/Bus26 ==
  Bus26 : powerlib/Measurements/Three-Phase V-I Measurement  VoltageMeasurement=no  SetLabelV=off  LabelV=Vabc  Vpu=off  VpuLL=off  CurrentMeasurement=no  SetLabelI=off  LabelI=Iabc  Ipu=off  Pbase=100e6  Vbase=500e3  OutputType=Complex  PhasorSimulation=off  PSBequivalent=0
  CB3-2 : powerlib/Elements/Three-Phase Breaker  InitialState=open  SwitchA=on  SwitchB=on  SwitchC=on  SwitchTimes="[1/60  5/60]"  External=off  BreakerResistance=0.01  SnubberResistance=1e6  SnubberCapacitance=inf  Measurements=None
  Load26 : powerlib/Elements/Three-Phase Series RLC Load  LConnTagsString=A|B|C  Configuration=Y (grounded)  NominalVoltage=1000  NominalFrequency=60  ActivePower=10e3  InductivePower=100  CapacitivePower=100  Measurements=None  LoadType=constant Z
  InPhaseA : PMIOPort  Port=1  Side=Left
  InPhaseB : PMIOPort  Port=2  Side=Left
  InPhaseC : PMIOPort  Port=3  Side=Left
  OutPhaseA : PMIOPort  Port=4  Side=Right
  OutPhaseB : PMIOPort  Port=5  Side=Right
  OutPhaseC : PMIOPort  Port=6  Side=Right
  connections:
  CB3-2/RConn3 -- OutPhaseC/RConn1
  Load26/LConn2 -- CB3-2/LConn2 -- Bus26/RConn2
  Bus26/RConn3 -- CB3-2/LConn3 -- Load26/LConn3
  CB3-2/RConn1 -- OutPhaseA/RConn1
  CB3-2/RConn2 -- OutPhaseB/RConn1
  Bus26/RConn1 -- CB3-2/LConn1 -- Load26/LConn1
  InPhaseA/RConn1 -- Bus26/LConn1
  InPhaseB/RConn1 -- Bus26/LConn2
  InPhaseC/RConn1 -- Bus26/LConn3

== system case33/Bus27 ==
  Bus27 : powerlib/Measurements/Three-Phase V-I Measurement  VoltageMeasurement=no  SetLabelV=off  LabelV=Vabc  Vpu=off  VpuLL=off  CurrentMeasurement=no  SetLabelI=off  LabelI=Iabc  Ipu=off  Pbase=100e6  Vbase=500e3  OutputType=Complex  PhasorSimulation=off  PSBequivalent=0
  CB3-2 : powerlib/Elements/Three-Phase Breaker  InitialState=open  SwitchA=on  SwitchB=on  SwitchC=on  SwitchTimes="[1/60  5/60]"  External=off  BreakerResistance=0.01  SnubberResistance=1e6  SnubberCapacitance=inf  Measurements=None
  Load27 : powerlib/Elements/Three-Phase Series RLC Load  LConnTagsString=A|B|C  Configuration=Y (grounded)  NominalVoltage=1000  NominalFrequency=60  ActivePower=10e3  InductivePower=100  CapacitivePower=100  Measurements=None  LoadType=constant Z
  InPhaseA : PMIOPort  Port=1  Side=Left
  InPhaseB : PMIOPort  Port=2  Side=Left
  InPhaseC : PMIOPort  Port=3  Side=Left
  OutPhaseA : PMIOPort  Port=4  Side=Right
  OutPhaseB : PMIOPort  Port=5  Side=Right
  OutPhaseC : PMIOPort  Port=6  Side=Right
  connections:
  CB3-2/LConn1 -- Load27/LConn1 -- Bus27/RConn1
  CB3-2/RConn3 -- OutPhaseC/RConn1
  CB3-2/LConn2 -- Load27/LConn2 -- Bus27/RConn2
  Bus27/RConn3 -- Load27/LConn3 -- CB3-2/LConn3
  CB3-2/RConn1 -- OutPhaseA/RConn1
  CB3-2/RConn2 -- OutPhaseB/RConn1
  InPhaseA/RConn1 -- Bus27/LConn1
  InPhaseB/RConn1 -- Bus27/LConn2
  InPhaseC/RConn1 -- Bus27/LConn3

== system case33/Bus28 ==
  Bus28 : powerlib/Measurements/Three-Phase V-I Measurement  VoltageMeasurement=no  SetLabelV=off  LabelV=Vabc  Vpu=off  VpuLL=off  CurrentMeasurement=no  SetLabelI=off  LabelI=Iabc  Ipu=off  Pbase=100e6  Vbase=500e3  OutputType=Complex  PhasorSimulation=off  PSBequivalent=0
  CB3-2 : powerlib/Elements/Three-Phase Breaker  InitialState=open  SwitchA=on  SwitchB=on  SwitchC=on  SwitchTimes="[1/60  5/60]"  External=off  BreakerResistance=0.01  SnubberResistance=1e6  SnubberCapacitance=inf  Measurements=None
  Load28 : powerlib/Elements/Three-Phase Series RLC Load  LConnTagsString=A|B|C  Configuration=Y (grounded)  NominalVoltage=1000  NominalFrequency=60  ActivePower=10e3  InductivePower=100  CapacitivePower=100  Measurements=None  LoadType=constant Z
  InPhaseA : PMIOPort  Port=1  Side=Left
  InPhaseB : PMIOPort  Port=2  Side=Left
  InPhaseC : PMIOPort  Port=3  Side=Left
  OutPhaseA : PMIOPort  Port=4  Side=Right
  OutPhaseB : PMIOPort  Port=5  Side=Right
  OutPhaseC : PMIOPort  Port=6  Side=Right
  connections:
  Load28/LConn1 -- CB3-2/LConn1 -- Bus28/RConn1
  CB3-2/RConn3 -- OutPhaseC/RConn1
  Load28/LConn2 -- CB3-2/LConn2 -- Bus28/RConn2
  Load28/LConn3 -- CB3-2/LConn3 -- Bus28/RConn3
  CB3-2/RConn1 -- OutPhaseA/RConn1
  CB3-2/RConn2 -- OutPhaseB/RConn1
  InPhaseA/RConn1 -- Bus28/LConn1
  InPhaseB/RConn1 -- Bus28/LConn2
  InPhaseC/RConn1 -- Bus28/LConn3

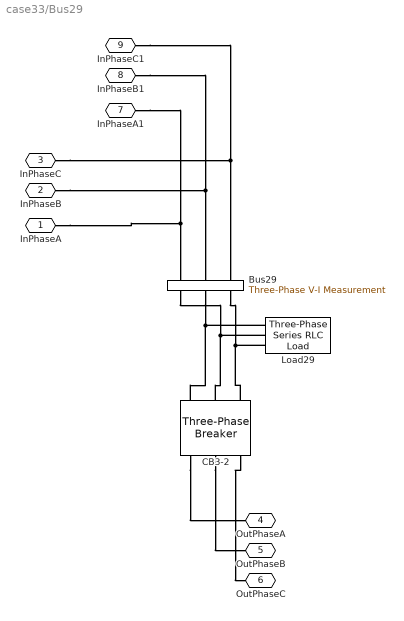
== system case33/Bus29 ==
  Bus29 : powerlib/Measurements/Three-Phase V-I Measurement  VoltageMeasurement=no  SetLabelV=off  LabelV=Vabc  Vpu=off  VpuLL=off  CurrentMeasurement=no  SetLabelI=off  LabelI=Iabc  Ipu=off  Pbase=100e6  Vbase=500e3  OutputType=Complex  PhasorSimulation=off  PSBequivalent=0
  CB3-2 : powerlib/Elements/Three-Phase Breaker  InitialState=open  SwitchA=on  SwitchB=on  SwitchC=on  SwitchTimes="[1/60  5/60]"  External=off  BreakerResistance=0.01  SnubberResistance=1e6  SnubberCapacitance=inf  Measurements=None
  Load29 : powerlib/Elements/Three-Phase Series RLC Load  LConnTagsString=A|B|C  Configuration=Y (grounded)  NominalVoltage=1000  NominalFrequency=60  ActivePower=10e3  InductivePower=100  CapacitivePower=100  Measurements=None  LoadType=constant Z
  InPhaseA : PMIOPort  Port=1  Side=Left
  InPhaseB : PMIOPort  Port=2  Side=Left
  InPhaseC : PMIOPort  Port=3  Side=Left
  OutPhaseA : PMIOPort  Port=4  Side=Right
  OutPhaseB : PMIOPort  Port=5  Side=Right
  OutPhaseC : PMIOPort  Port=6  Side=Right
  InPhaseA1 : PMIOPort  Port=7  Side=Left
  InPhaseB1 : PMIOPort  Port=8  Side=Left
  InPhaseC1 : PMIOPort  Port=9  Side=Left
  connections:
  Bus29/RConn1 -- CB3-2/LConn1 -- Load29/LConn1
  CB3-2/RConn3 -- OutPhaseC/RConn1
  Load29/LConn2 -- CB3-2/LConn2 -- Bus29/RConn2
  Load29/LConn3 -- CB3-2/LConn3 -- Bus29/RConn3
  CB3-2/RConn1 -- OutPhaseA/RConn1
  CB3-2/RConn2 -- OutPhaseB/RConn1
  InPhaseB1/RConn1 -- InPhaseB/RConn1 -- Bus29/LConn2
  InPhaseA1/RConn1 -- InPhaseA/RConn1 -- Bus29/LConn1
  InPhaseC1/RConn1 -- InPhaseC/RConn1 -- Bus29/LConn3

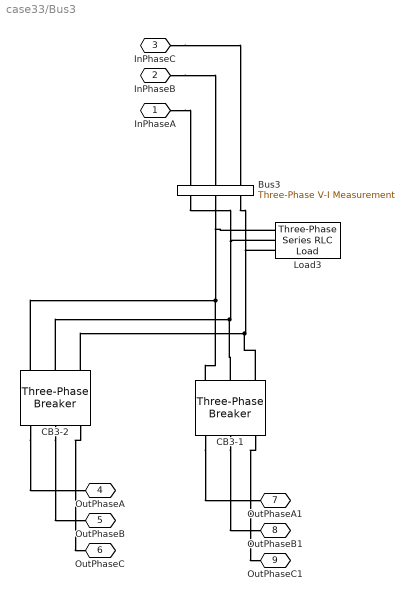
== system case33/Bus3 ==
  Bus3 : powerlib/Measurements/Three-Phase V-I Measurement  VoltageMeasurement=no  SetLabelV=off  LabelV=Vabc  Vpu=off  VpuLL=off  CurrentMeasurement=no  SetLabelI=off  LabelI=Iabc  Ipu=off  Pbase=100e6  Vbase=500e3  OutputType=Complex  PhasorSimulation=off  PSBequivalent=0
  CB3-1 : powerlib/Elements/Three-Phase Breaker  InitialState=open  SwitchA=on  SwitchB=on  SwitchC=on  SwitchTimes="[1/60  5/60]"  External=off  BreakerResistance=0.01  SnubberResistance=1e6  SnubberCapacitance=inf  Measurements=None
  CB3-2 : powerlib/Elements/Three-Phase Breaker  InitialState=open  SwitchA=on  SwitchB=on  SwitchC=on  SwitchTimes="[1/60  5/60]"  External=off  BreakerResistance=0.01  SnubberResistance=1e6  SnubberCapacitance=inf  Measurements=None
  Load3 : powerlib/Elements/Three-Phase Series RLC Load  LConnTagsString=A|B|C  Configuration=Y (grounded)  NominalVoltage=1000  NominalFrequency=60  ActivePower=10e3  InductivePower=100  CapacitivePower=100  Measurements=None  LoadType=constant Z
  InPhaseA : PMIOPort  Port=1  Side=Left
  InPhaseB : PMIOPort  Port=2  Side=Left
  InPhaseC : PMIOPort  Port=3  Side=Left
  OutPhaseA : PMIOPort  Port=4  Side=Right
  OutPhaseB : PMIOPort  Port=5  Side=Right
  OutPhaseC : PMIOPort  Port=6  Side=Right
  OutPhaseA1 : PMIOPort  Port=7  Side=Right
  OutPhaseB1 : PMIOPort  Port=8  Side=Right
  OutPhaseC1 : PMIOPort  Port=9  Side=Right
  connections:
  CB3-2/LConn1 -- CB3-1/LConn1 -- Load3/LConn1 -- Bus3/RConn1
  CB3-2/RConn3 -- OutPhaseC/RConn1
  CB3-1/LConn2 -- Load3/LConn2 -- Bus3/RConn2 -- CB3-2/LConn2
  CB3-1/LConn3 -- Bus3/RConn3 -- Load3/LConn3 -- CB3-2/LConn3
  CB3-2/RConn1 -- OutPhaseA/RConn1
  CB3-2/RConn2 -- OutPhaseB/RConn1
  CB3-1/RConn3 -- OutPhaseC1/RConn1
  CB3-1/RConn1 -- OutPhaseA1/RConn1
  CB3-1/RConn2 -- OutPhaseB1/RConn1
  InPhaseA/RConn1 -- Bus3/LConn1
  InPhaseB/RConn1 -- Bus3/LConn2
  InPhaseC/RConn1 -- Bus3/LConn3

== system case33/Bus30 ==
  Bus30 : powerlib/Measurements/Three-Phase V-I Measurement  VoltageMeasurement=no  SetLabelV=off  LabelV=Vabc  Vpu=off  VpuLL=off  CurrentMeasurement=no  SetLabelI=off  LabelI=Iabc  Ipu=off  Pbase=100e6  Vbase=500e3  OutputType=Complex  PhasorSimulation=off  PSBequivalent=0
  CB3-2 : powerlib/Elements/Three-Phase Breaker  InitialState=open  SwitchA=on  SwitchB=on  SwitchC=on  SwitchTimes="[1/60  5/60]"  External=off  BreakerResistance=0.01  SnubberResistance=1e6  SnubberCapacitance=inf  Measurements=None
  Load30 : powerlib/Elements/Three-Phase Series RLC Load  LConnTagsString=A|B|C  Configuration=Y (grounded)  NominalVoltage=1000  NominalFrequency=60  ActivePower=10e3  InductivePower=100  CapacitivePower=100  Measurements=None  LoadType=constant Z
  InPhaseA : PMIOPort  Port=1  Side=Left
  InPhaseB : PMIOPort  Port=2  Side=Left
  InPhaseC : PMIOPort  Port=3  Side=Left
  OutPhaseA : PMIOPort  Port=4  Side=Right
  OutPhaseB : PMIOPort  Port=5  Side=Right
  OutPhaseC : PMIOPort  Port=6  Side=Right
  connections:
  Bus30/RConn1 -- CB3-2/LConn1 -- Load30/LConn1
  CB3-2/RConn3 -- OutPhaseC/RConn1
  Load30/LConn2 -- CB3-2/LConn2 -- Bus30/RConn2
  Load30/LConn3 -- CB3-2/LConn3 -- Bus30/RConn3
  CB3-2/RConn1 -- OutPhaseA/RConn1
  CB3-2/RConn2 -- OutPhaseB/RConn1
  InPhaseB/RConn1 -- Bus30/LConn2
  InPhaseA/RConn1 -- Bus30/LConn1
  InPhaseC/RConn1 -- Bus30/LConn3

== system case33/Bus31 ==
  Bus31 : powerlib/Measurements/Three-Phase V-I Measurement  VoltageMeasurement=no  SetLabelV=off  LabelV=Vabc  Vpu=off  VpuLL=off  CurrentMeasurement=no  SetLabelI=off  LabelI=Iabc  Ipu=off  Pbase=100e6  Vbase=500e3  OutputType=Complex  PhasorSimulation=off  PSBequivalent=0
  CB3-2 : powerlib/Elements/Three-Phase Breaker  InitialState=open  SwitchA=on  SwitchB=on  SwitchC=on  SwitchTimes="[1/60  5/60]"  External=off  BreakerResistance=0.01  SnubberResistance=1e6  SnubberCapacitance=inf  Measurements=None
  Load31 : powerlib/Elements/Three-Phase Series RLC Load  LConnTagsString=A|B|C  Configuration=Y (grounded)  NominalVoltage=1000  NominalFrequency=60  ActivePower=10e3  InductivePower=100  CapacitivePower=100  Measurements=None  LoadType=constant Z
  InPhaseA : PMIOPort  Port=1  Side=Left
  InPhaseB : PMIOPort  Port=2  Side=Left
  InPhaseC : PMIOPort  Port=3  Side=Left
  OutPhaseA : PMIOPort  Port=4  Side=Right
  OutPhaseB : PMIOPort  Port=5  Side=Right
  OutPhaseC : PMIOPort  Port=6  Side=Right
  connections:
  Bus31/RConn1 -- CB3-2/LConn1 -- Load31/LConn1
  CB3-2/RConn3 -- OutPhaseC/RConn1
  Load31/LConn2 -- CB3-2/LConn2 -- Bus31/RConn2
  Load31/LConn3 -- CB3-2/LConn3 -- Bus31/RConn3
  CB3-2/RConn1 -- OutPhaseA/RConn1
  CB3-2/RConn2 -- OutPhaseB/RConn1
  InPhaseA/RConn1 -- Bus31/LConn1
  Bus31/LConn2 -- InPhaseB/RConn1
  InPhaseC/RConn1 -- Bus31/LConn3

== system case33/Bus32 ==
  Bus32 : powerlib/Measurements/Three-Phase V-I Measurement  VoltageMeasurement=no  SetLabelV=off  LabelV=Vabc  Vpu=off  VpuLL=off  CurrentMeasurement=no  SetLabelI=off  LabelI=Iabc  Ipu=off  Pbase=100e6  Vbase=500e3  OutputType=Complex  PhasorSimulation=off  PSBequivalent=0
  CB3-2 : powerlib/Elements/Three-Phase Breaker  InitialState=open  SwitchA=on  SwitchB=on  SwitchC=on  SwitchTimes="[1/60  5/60]"  External=off  BreakerResistance=0.01  SnubberResistance=1e6  SnubberCapacitance=inf  Measurements=None
  Load32 : powerlib/Elements/Three-Phase Series RLC Load  LConnTagsString=A|B|C  Configuration=Y (grounded)  NominalVoltage=1000  NominalFrequency=60  ActivePower=10e3  InductivePower=100  CapacitivePower=100  Measurements=None  LoadType=constant Z
  InPhaseA : PMIOPort  Port=1  Side=Left
  InPhaseB : PMIOPort  Port=2  Side=Left
  InPhaseC : PMIOPort  Port=3  Side=Left
  OutPhaseA : PMIOPort  Port=4  Side=Right
  OutPhaseB : PMIOPort  Port=5  Side=Right
  OutPhaseC : PMIOPort  Port=6  Side=Right
  connections:
  Bus32/RConn1 -- CB3-2/LConn1 -- Load32/LConn1
  CB3-2/RConn3 -- OutPhaseC/RConn1
  Load32/LConn2 -- CB3-2/LConn2 -- Bus32/RConn2
  Bus32/RConn3 -- Load32/LConn3 -- CB3-2/LConn3
  CB3-2/RConn1 -- OutPhaseA/RConn1
  CB3-2/RConn2 -- OutPhaseB/RConn1
  InPhaseA/RConn1 -- Bus32/LConn1
  InPhaseB/RConn1 -- Bus32/LConn2
  InPhaseC/RConn1 -- Bus32/LConn3
